simulink model "model2_disc"  (R2021b)
settings: Solver=VariableStepAuto  StartTime=0.0  StopTime=100  RelTol=1e-3
values from neighbouring files (symbols this model uses):
  H_disc = c2d(H_lin, Te, 'tustin')    [proiectMS.m]
undefined symbols (not defined in the file or in its folder): C_disc, D_disc, ustarr, xstarr, ystarr
settings Model: Creator=AMY  LastModifiedBy=AMY

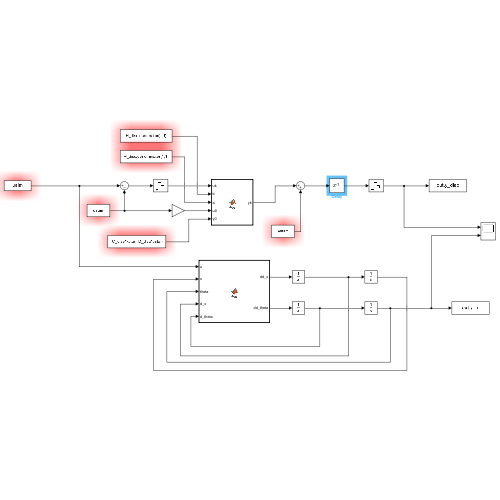
[thumbnail: Simulink's stored preview of the top-level diagram]
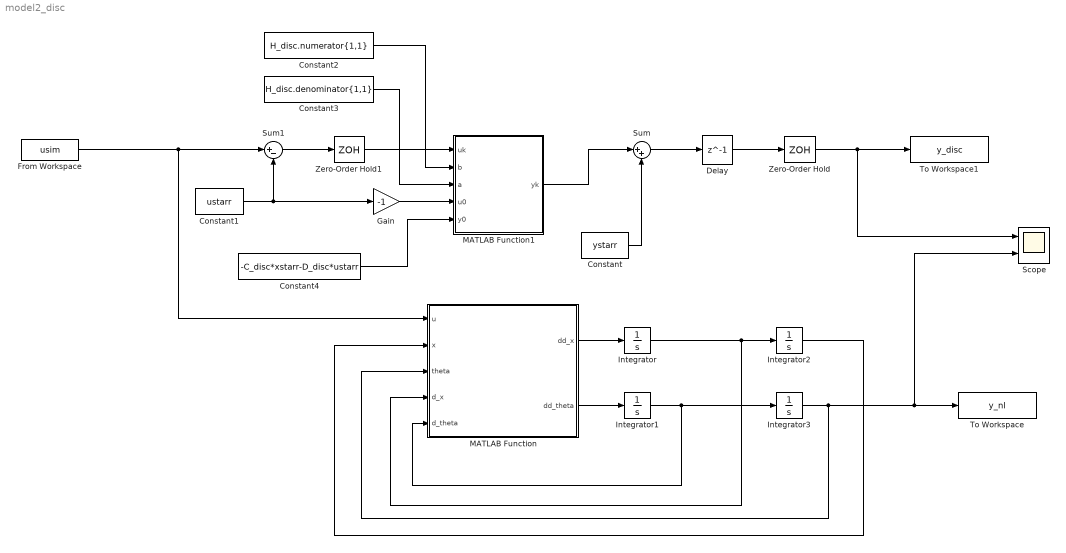
== system model2_disc ==
  Constant : Constant  Value=ystarr
  Constant1 : Constant  Value=ustarr
  Constant2 : Constant  Value=H_disc.numerator{1,1}
  Constant3 : Constant  Value=H_disc.denominator{1,1}
  Constant4 : Constant  Value=-C_disc*xstarr-D_disc*ustarr
  Delay : Delay  DelayLength=1  SampleTime=0.09
  From Workspace : FromWorkspace  VariableName=usim
  Gain : Gain  Gain=-1
  Integrator{,1..3} (4 alike) : Integrator
  MATLAB Function : MATLAB Function  TreatAsAtomicUnit=on
  MATLAB Function1 : MATLAB Function  TreatAsAtomicUnit=on
  Scope : Scope  NumInputPorts=2
  Sum : Sum  Inputs=|++
  Sum1 : Sum  Inputs=|+-
  To Workspace : ToWorkspace  VariableName=y_nl  SaveFormat=Timeseries  SampleTime=-1
      settings: Save2DSignal=2-D array (concatenate along first dimension)
  To Workspace1 : ToWorkspace  VariableName=y_disc  SaveFormat=Timeseries  SampleTime=-1
      settings: Save2DSignal=2-D array (concatenate along first dimension)
  Zero-Order Hold : ZeroOrderHold  SampleTime=-1
  Zero-Order Hold1 : ZeroOrderHold  SampleTime=-1
  wires:
  Integrator1/1 -> Integrator3/1, MATLAB Function/5(d_theta)
  Integrator/1 -> MATLAB Function/4(d_x), Integrator2/1
  From Workspace/1 -> Sum1/1, MATLAB Function/1(u)
  Integrator3/1 -> Scope/2, To Workspace/1, MATLAB Function/3(theta)
  MATLAB Function/2(dd_theta) -> Integrator1/1
  Integrator2/1 -> MATLAB Function/2(x)
  MATLAB Function/1(dd_x) -> Integrator/1
  MATLAB Function1/1(yk) -> Sum/1
  Constant/1 -> Sum/2
  Sum/1 -> Delay/1
  Delay/1 -> Zero-Order Hold/1
  Zero-Order Hold/1 -> Scope/1, To Workspace1/1
  Zero-Order Hold1/1 -> MATLAB Function1/1(uk)
  Sum1/1 -> Zero-Order Hold1/1
  Constant1/1 -> Sum1/2, Gain/1
  Gain/1 -> MATLAB Function1/4(u0)
  Constant2/1 -> MATLAB Function1/2(b)
  Constant3/1 -> MATLAB Function1/3(a)
  Constant4/1 -> MATLAB Function1/5(y0)

== matlab function model2_disc/MATLAB Function1 ==
  data: yk output; uk input; b input; a input; u0 input; y0 input
function yk  = fcn(uk, b, a,  u0, y0)

    persistent uk1
    persistent uk2
    persistent uk3
    persistent uk4
    persistent yk1
    persistent yk2
    persistent yk3
    persistent yk4

    %Coeficientii numaratorului functiei de transfer discrete
    b0 = b(1);
    b1 = b(2);
    b2 = b(3);
    b3 = b(4);
    b4 = b(5);

    %Coeficientii numaratorului functiei de transfer discrete
    a0 = a(1);
    a1 = a(2);
    a2 = a(3);
    a3 = a(4);
    a4 = a(5);

    if (isempty(uk1) && isempty(uk2) && isempty(uk3) && isempty(uk4) && isempty(yk1) && isempty(yk2) && isempty(yk3) && isempty(yk4))
        uk1 = u0;
        uk2 = u0;
        uk3 = u0;
        uk4 = u0;
        yk1 = y0;
        yk2 = y0;
        yk3 = y0;
        yk4 = y0;
    end

    %Relatia de recurenta
    yk = (1/a0)*(b0*uk + b1*uk1 + b2*uk2 + b3*uk3 + b4*uk4 - a1*yk1 - a2*yk2 - a3*yk3 - a4*yk4);

    %Actualizarea valorilor
    yk4 = yk3;
    yk3 = yk2;
    yk2 = yk1;
    yk1 = yk;
    uk4 = uk3;
    uk3 = uk2;
    uk2 = uk1;
    uk1 = uk;

end

== matlab function model2_disc/MATLAB Function ==
  data: dd_x output; u input; dd_theta output; x input; theta input; d_x input; d_theta input
function [dd_x, dd_theta] = fcn(u, x, theta,  d_x, d_theta)

    m = 1.5;          %Masa corpului
    g = 9.81;         %Acceleratia gravitationala
    zeta = 0.6;      %Coeficient de amortizare
    k = 1.5;          %Constanta elastica
    l0 = 0.5;         %Lungimea initiala a resortului
    
    %Ecuatiile
    dd_x = (l0+x)*(d_theta)*(d_theta) - (k/m)*x + g*cos(theta) - zeta*d_x;
    dd_theta = -(g/(l0+x)*sin(theta))-(2*d_x/(l0+x))*d_theta - zeta*d_theta + 1/(m*(l0+x)*(l0+x))*u;

end
